simulink model "linear_system"  (R2018b)
settings: Solver=VariableStepAuto  StartTime=0.0  StopTime=50.0  RelTol=1e-3
settings Model: Creator=saramohamadi  LastModifiedBy=aniruddhgp

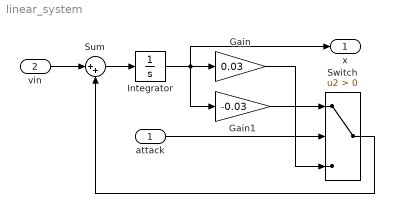
== system linear_system ==
  attack : Inport
  vin : Inport  Port=2
  Gain : Gain  Gain=0.03
  Gain1 : Gain  Gain=-0.03
  Integrator : Integrator  InitialCondition=1
  Sum : Sum  Inputs=|++
  Switch : Switch  Criteria=u2 > Threshold
  x : Outport
  wires:
  Gain/1 -> Switch/3
  Sum/1 -> Integrator/1
  Gain1/1 -> Switch/1
  vin/1 -> Sum/1
  Switch/1 -> Sum/2
  Integrator/1 -> x/1, Gain1/1, Gain/1
  attack/1 -> Switch/2
